simulink model "fir_filter_model"  (R2019b)
settings: Solver=FixedStepAuto  StartTime=0.0  StopTime=length(x)-1  RelTol=1e-3
model workspace (MAT data in the model file):
  T.input = []
  T.output = []
  T.sum = []
  T.coefficient = []
  T.index = []
  b = [-0.000630469148644 -0.00181856812428 -0.00256194161246 -0.0015874939944 0.00236951266897 0.00833249697835 0.011803612855 0.00675929677933 -0.00917451199773 -0.029730906886 -0.0398164522664 -0.0223016476387 0.0310279659072 0.111143500493 0.192455402101 0.243730203886 0.243730203886 0.192455402101 0.111143500493 0.0310279659072 -0.0223016476387 -0.0398164522664 -0.029730906886 -0.00917451199773 0.00675929677933 0.011803612855 0.00833249697835 0.00236951266897 -0.0015874939944 -0.00256194161246 -0.00181856812428 -0.000630469148644]
  x = [0 0.00314158748588 0.0125660398834 0.0282705667703 0.0502443181798 0.0784590957278 0.112856384873 0.153330783737 0.199709980514 0.251731548668 0.309016994375 0.371043710237 ... (411 elements, 411x1)]
values from neighbouring files (symbols this model uses):
  T = fir_filter_double_types    [test_matlab_function_block.m]
libraries: dspsrcs4 x1
settings Model: Creator=tbryan  LastModifiedBy=tbryan
settings HardwareCC: ProdBitPerLong=64  ProdHWDeviceType=Intel->x86-64 (Mac OS X)
settings SFSimCC: SimParseCustomCode=off

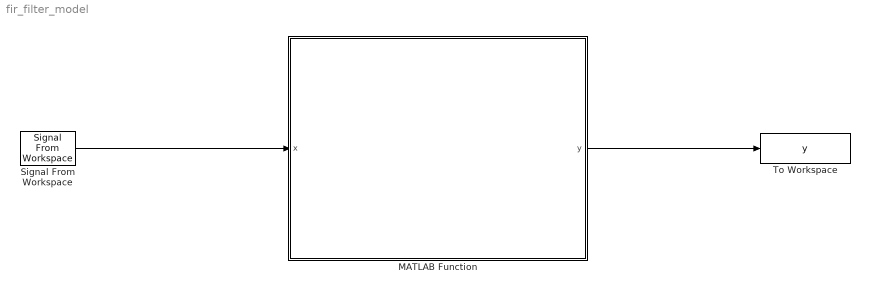
== system fir_filter_model ==
  MATLAB Function : MATLAB Function  TreatAsAtomicUnit=on
  Signal From Workspace : dspsrcs4/Signal From Workspace  X=x  Ts=1  nsamps=1  OutputAfterFinalValue=Setting to zero  ignoreOrWarnInputAndFrameLengths=off  OutputFrames=off
  To Workspace : ToWorkspace  VariableName=y  SampleTime=-1
  wires:
  Signal From Workspace/1 -> MATLAB Function/1(x)
  MATLAB Function/1(y) -> To Workspace/1

== matlab function fir_filter_model/MATLAB Function ==
  data: x input; y output; b parameter; T parameter
function y = fir_filter_matlab_function_block(x,b,T)
    persistent z
    persistent p
    if isempty(z)
        z = zeros(size(b),'like',T.input);
        p = cast(0,'like',T.index);
    end
    %[y,z,p] = fir_filter(b,x,z,p,T);
    [y,z,p] = fir_filter(b,x,z,p);
end
